simulink model "follower"  (R2020b)
settings: Solver=VariableStepAuto  StartTime=0.0  StopTime=10.0  RelTol=1e-3
libraries: simulink x5, uavalgslib x2
settings Model: Creator=USER  LastModifiedBy=USER

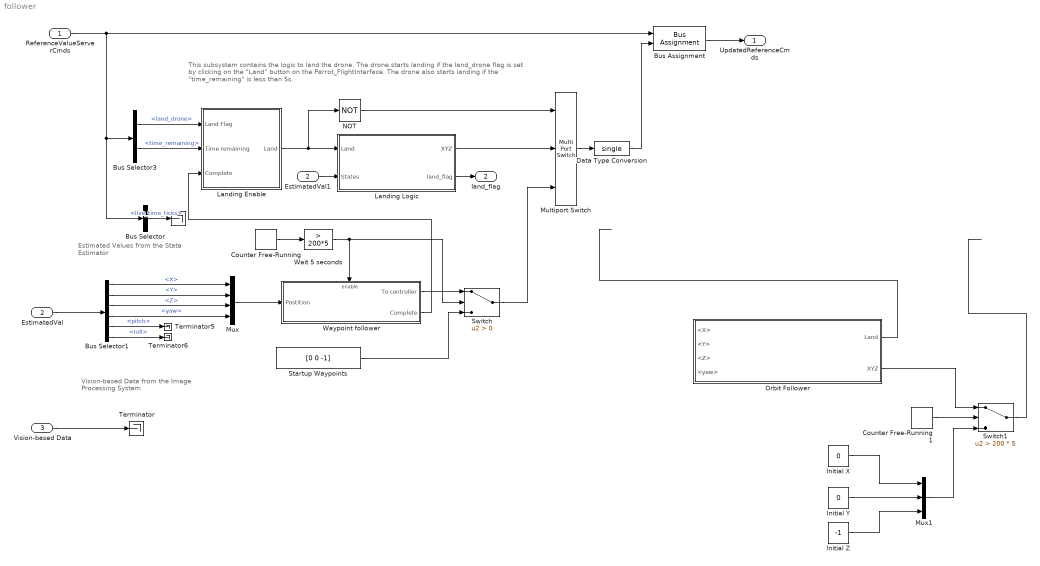
== system follower ==
  note: Estimated Values from the
      | State Estimator
  note: Vision-based Data from the
      | Image Processing System
  note: This subsystem contains the logic to land the drone. The drone starts landing if the
      | land_drone flag is set by clicking on the  "Land" button on the Parrot_FlightInterface.
      | The drone also starts landing if the "time_remaining" is less than 5s.
  ReferenceValueServerCmds : Inport
  EstimatedVal : Inport  Port=2
  Vision-based Data : Inport  Port=3
  " " : Terminator
  Bus Selector : BusSelector  OutputSignals=live_time_ticks
  Bus Selector1 : BusSelector  OutputSignals=X,Y,Z,yaw,pitch,roll
  Bus Selector3 : BusSelector  OutputSignals=land_drone,time_remaining
  Bus Assignment : BusAssignment  AssignedSignals=pos_ref
  Counter Free-Running : simulink/Sources/Counter Free-Running  NumBits=32  tsamp=-1
  Counter Free-Running1 : simulink/Sources/Counter Free-Running  NumBits=32  tsamp=-1
  Data Type Conversion : DataTypeConversion  OutDataTypeStr=single
  EstimatedVal1 : InportShadow  Port=2
  Initial X : Constant  Value=0  OutDataTypeStr=single
  Initial Y : Constant  Value=0  OutDataTypeStr=single
  Initial Z : Constant  Value=-1  OutDataTypeStr=single
  Landing Enable : Subsystem
  Landing Logic : Subsystem
  Multiport Switch : MultiPortSwitch  DataPortOrder=Zero-based contiguous  Inputs=2  zeroidx=on
  Mux : Mux
  Mux1 : Mux  Inputs=3
  NOT : Logic  Operator=NOT  IconShape=distinctive  AllPortsSameDT=off  OutDataTypeStr=boolean
  Orbit Follower : Subsystem
  Startup Waypoints : Constant  Value=[0 0 -1]
  Switch : Switch  Criteria=u2 > Threshold
  Switch1 : Switch  Criteria=u2 > Threshold  Threshold=200 * 5
  Terminator : Terminator
  Terminator5 : Terminator
  Terminator6 : Terminator
  Wait 5 seconds : simulink/Logic and Bit Operations/Compare To Constant  relop=>  const=200*5  OutDataTypeStr=boolean
  Waypoint follower : Subsystem
  UpdatedReferenceCmds : Outport  VectorParamsAs1DForOutWhenUnconnected=off
  land_flag : Outport  Port=2
  wires:
  Waypoint follower/2(Complete) -> Landing Enable/3(Complete)
  Bus Assignment/1 -> UpdatedReferenceCmds/1
  Bus Selector3/2 -> Landing Enable/2(Time remaining)  "<time_remaining>"
  Landing Enable/1(Land) -> NOT/1, Landing Logic/1(Land)
  Mux/1 -> Waypoint follower/1(Postition)
  Bus Selector1/5 -> Terminator5/1  "<pitch>"
  Bus Selector1/2 -> Mux/2  "<Y>"
  Data Type Conversion/1 -> Bus Assignment/2
  Landing Logic/1(XYZ) -> Multiport Switch/2
  Multiport Switch/1 -> Data Type Conversion/1
  Startup Waypoints/1 -> Switch/3
  Landing Logic/2(land_flag) -> land_flag/1
  Bus Selector3/1 -> Landing Enable/1(Land Flag)  "<land_drone>"
  Bus Selector1/3 -> Mux/3  "<Z>"
  Bus Selector/1 -> " "/1  "<live_time_ticks>"
  ReferenceValueServerCmds/1 -> Bus Selector/1, Bus Selector3/1, Bus Assignment/1
  Switch/1 -> Multiport Switch/3
  NOT/1 -> Multiport Switch/1
  Vision-based Data/1 -> Terminator/1
  Bus Selector1/4 -> Mux/4  "<yaw>"
  Bus Selector1/1 -> Mux/1  "<X>"
  Counter Free-Running/1 -> Wait 5 seconds/1
  EstimatedVal/1 -> Bus Selector1/1
  Wait 5 seconds/1 -> Waypoint follower/Enable, Switch/2
  Waypoint follower/1(To controller) -> Switch/1
  Bus Selector1/6 -> Terminator6/1  "<roll>"
  EstimatedVal1/1 -> Landing Logic/2(States)
  Mux1/1 -> Switch1/3
  Initial Z/1 -> Mux1/3
  Switch1/1 -> ?
  Counter Free-Running1/1 -> Switch1/2
  Initial Y/1 -> Mux1/2
  Orbit Follower/2(XYZ) -> Switch1/1
  Initial X/1 -> Mux1/1
  ? -> Orbit Follower/3(<Z>)  "<Z>"
  ? -> Orbit Follower/4(<yaw>)  "<yaw>"
  ? -> Orbit Follower/2(<Y>)  "<Y>"
  Orbit Follower/1(Land) -> ?
  ? -> Orbit Follower/1(<X>)  "<X>"

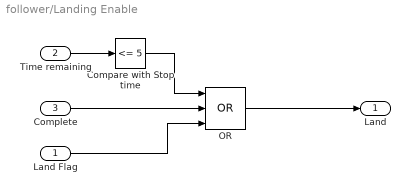
== system follower/Landing Enable ==
  Land Flag : Inport
  Time remaining : Inport  Port=2
  Complete : Inport  Port=3
  Compare with Stop time : simulink/Logic and Bit Operations/Compare To Constant  relop=<=  const=5  OutDataTypeStr=boolean
  OR : Logic  Operator=OR  Inputs=3  IconShape=distinctive  AllPortsSameDT=off  OutDataTypeStr=boolean
  Land : Outport
  wires:
  Compare with Stop time/1 -> OR/1
  Time remaining/1 -> Compare with Stop time/1
  Land Flag/1 -> OR/3
  OR/1 -> Land/1
  Complete/1 -> OR/2

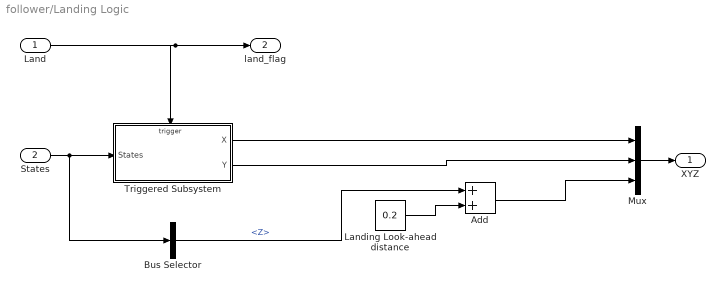
== system follower/Landing Logic ==
  Land : Inport
  States : Inport  Port=2
  Add : Sum
  Bus Selector : BusSelector  OutputSignals=Z
  Landing Look-ahead distance : Constant  Value=0.2  OutDataTypeStr=single
  Mux : Mux  Inputs=3
  Triggered Subsystem : Subsystem  TreatAsAtomicUnit=on
  XYZ : Outport
  land_flag : Outport  Port=2
  wires:
  States/1 -> Bus Selector/1, Triggered Subsystem/1(States)
  Mux/1 -> XYZ/1
  Add/1 -> Mux/3
  Landing Look-ahead distance/1 -> Add/2
  Triggered Subsystem/1(X) -> Mux/1
  Triggered Subsystem/2(Y) -> Mux/2
  Bus Selector/1 -> Add/1  "<Z>"
  Land/1 -> land_flag/1, Triggered Subsystem/Trigger

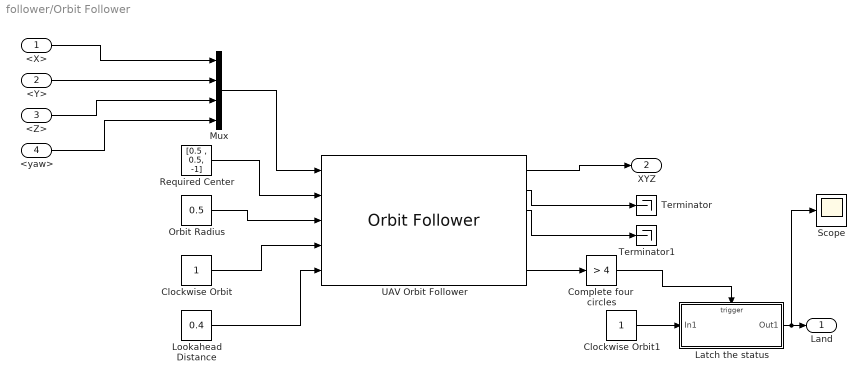
== system follower/Orbit Follower ==
  <X> : Inport
  <Y> : Inport  Port=2
  <Z> : Inport  Port=3
  <yaw> : Inport  Port=4
  Clockwise Orbit : Constant  OutDataTypeStr=single
  Clockwise Orbit1 : Constant  OutDataTypeStr=single
  "Complete four  circles " : simulink/Logic and Bit Operations/Compare To Constant  relop=>  const=4  OutDataTypeStr=boolean
  Latch the status : Subsystem  TreatAsAtomicUnit=on
  Lookahead Distance : Constant  Value=0.4  OutDataTypeStr=single
  Mux : Mux
  Orbit Radius : Constant  Value=0.5  OutDataTypeStr=single
  Required Center : Constant  Value="[0.5 ,  0.5, -1]"  OutDataTypeStr=single
  Scope : Scope
  Terminator : Terminator
  Terminator1 : Terminator
  UAV Orbit Follower : uavalgslib/Orbit Follower  UAVType=multirotor  MinOrbitRadius=1  MinLookaheadDistance=0.1  ExternalReset=none  ShowCrossTrackErrorOutput=off  ShowNumTurnsOutput=on  SimulateUsing=Interpreted execution
      settings: SourceProductName=UAV Toolbox
  Land : Outport
  XYZ : Outport  Port=2
  wires:
  <Y>/1 -> Mux/2
  Required Center/1 -> UAV Orbit Follower/2
  Mux/1 -> UAV Orbit Follower/1
  UAV Orbit Follower/2 -> Terminator/1
  Lookahead Distance/1 -> UAV Orbit Follower/5
  UAV Orbit Follower/1 -> XYZ/1
  <X>/1 -> Mux/1
  Orbit Radius/1 -> UAV Orbit Follower/3
  UAV Orbit Follower/3 -> Terminator1/1
  <Z>/1 -> Mux/3
  <yaw>/1 -> Mux/4
  Clockwise Orbit/1 -> UAV Orbit Follower/4
  Latch the status/1(Out1) -> Scope/1, Land/1
  "Complete four  circles "/1 -> Latch the status/Trigger
  Clockwise Orbit1/1 -> Latch the status/1(In1)
  UAV Orbit Follower/6 -> "Complete four  circles "/1

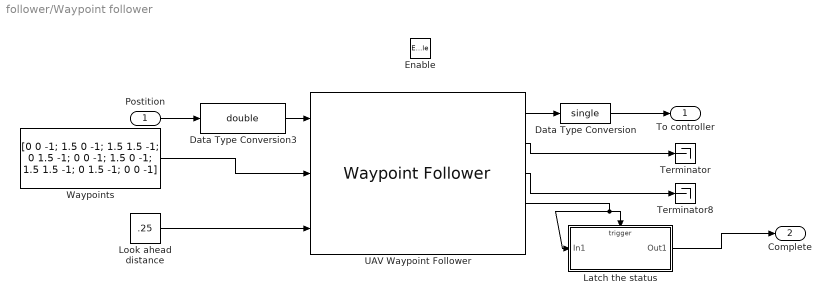
== system follower/Waypoint follower ==
  Postition : Inport
  Enable : EnablePort
  Data Type Conversion : DataTypeConversion  OutDataTypeStr=single
  Data Type Conversion3 : DataTypeConversion  OutDataTypeStr=double
  Latch the status : Subsystem  TreatAsAtomicUnit=on
  Look ahead distance : Constant  Value=.25  SampleTime=-1
  Terminator : Terminator
  Terminator8 : Terminator
  UAV Waypoint Follower : uavalgslib/Waypoint Follower  UAVType=multirotor  StartFrom=first  TransitionRadiusSource=internal  TransitionRadius=.3  MinLookaheadDistance=0.1  YawInput=off  ShowCrossTrackErrorOutput=off  ShowStatusOutput=on  SimulateUsing=Interpreted execution
      settings: SourceProductName=UAV Toolbox
  Waypoints : Constant  Value=[0 0 -1; 1.5 0 -1; 1.5 1.5 -1; 0 1.5 -1; 0 0 -1; 1.5 0 -1; 1.5 1.5 -1; 0 1.5 -1; 0 0 -1]  SampleTime=-1
  To controller : Outport  VectorParamsAs1DForOutWhenUnconnected=off
  Complete : Outport  Port=2
  wires:
  UAV Waypoint Follower/1 -> Data Type Conversion/1
  UAV Waypoint Follower/3 -> Terminator8/1
  Postition/1 -> Data Type Conversion3/1
  Waypoints/1 -> UAV Waypoint Follower/2
  UAV Waypoint Follower/2 -> Terminator/1
  Data Type Conversion/1 -> To controller/1
  Look ahead distance/1 -> UAV Waypoint Follower/3
  Data Type Conversion3/1 -> UAV Waypoint Follower/1
  UAV Waypoint Follower/4 -> Latch the status/1(In1), Latch the status/Trigger
  Latch the status/1(Out1) -> Complete/1

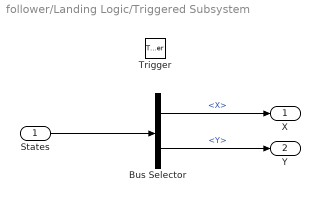
== system follower/Landing Logic/Triggered Subsystem ==
  States : Inport
  Trigger : TriggerPort  VariantControl=Variant  InitialTriggerSignalState=zero
  Bus Selector : BusSelector  OutputSignals=X,Y
  X : Outport
  Y : Outport  Port=2
  wires:
  States/1 -> Bus Selector/1
  Bus Selector/1 -> X/1  "<X>"
  Bus Selector/2 -> Y/1  "<Y>"

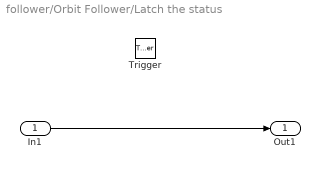
== system follower/Orbit Follower/Latch the status ==
  In1 : Inport
  Trigger : TriggerPort  VariantControl=Variant
  Out1 : Outport
  wires:
  In1/1 -> Out1/1

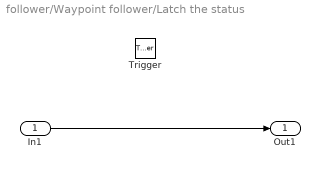
== system follower/Waypoint follower/Latch the status ==
  In1 : Inport
  Trigger : TriggerPort  VariantControl=Variant
  Out1 : Outport
  wires:
  In1/1 -> Out1/1
